simulink library "pv_sapm"  (R2018b)
settings: Solver=VariableStepAuto  StartTime=0.0  StopTime=10.0  RelTol=1e-3
undefined symbols (not defined in the file): Davies, Hay, path_carnot
libraries: carnot x4
settings Model: Creator=P41573  LastModifiedBy=P41573
settings SFSimCC: SimUseLocalCustomCode=off
settings RTWCC: RTWUseLocalCustomCode=off
settings CodeAppCC: StateflowObjectComments=on

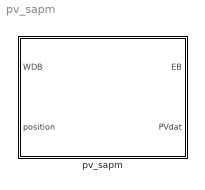
== system pv_sapm ==
  pv_sapm : Subsystem  mask(configurated PV Panel){PathName=fullfile(path_carnot('libsl'), 'Source', 'Electric_Generator', 'Pv_Sapm', 'parameter_set'), FileName='SandiaModuleDatabase.mat', Module=Yingli Solar YL230-29b Module - Sandia measured, userPath=on, userParam=off, Isco=8.222, Impo=7.727, Vmpo=29.886, Voco=37.28, T0=25, aIsc=0.000746, aImp=0.000176, BVoco=-0.1294, BVmpo=-0.137, n=1.263, SeriesCells=60, mBVoc=0, mBVmp=0, Ixo=8.1509, Ixxo=5.5099, C0=0.9993, C1=0.0007, C2=-0.058706, C3=-8.35334, C4=0.995, C5=0.005, C6=1.1325, C7=-0.1325, KbAngles=[0:5:90], Kb=[1 1 0.9999 0.9996 0.9991 0.9982 0.9965 0.9935 0.9886 0.9807 0.9678 0.9473 0.9148 0.8638 0.7846 0.6644 0.4907 0.2599 0], Kd=0.91, TypeMount=<propagated>, E0=1000, dTc=3, a=-3.348, b=-0.09143, TimeConstant=300, tini=20, ms=1, mp=1}
      mask prompts: PathName "Path"; FileName "DataBase"; Module "Parameter Set"; userPath "Edit path and name of parameter set"; userParam "User defined parameters"; Isco "reference short circuit current [A]"; Impo "reference maximum power point current [A]"; Vmpo "reference maximum power point voltage [V]"; Voco "reference open circuit voltage [V]"; T0 "reference cell temperature [°C]"; aIsc "temperature coef. for Isc [1/K]"; aImp "temperature coeff. for Imp [1/K]"; BVoco "temperature coef. for Voc [V/K]"; BVmpo "temperature coef. for Vmp [V/K]"; n "diode factor [n]"; SeriesCells "number of cells in series [-]"; mBVoc "irradiance dependant temperature coef. for Voc [V/K.wm2]"; mBVmp "irradiance dependant temperature coef. for Vmp [V/K.wm2]"; Ixo "Ix0 [A]"; Ixxo "Ixx0 [A]"; KbAngles "Kb: angles for longitudinal and transversal IAM [degree]"; Kb "Kb : incident angle modifier beam radiation"; Kd "Kd : Incidence angle modifier diffuse radiation"; TypeMount "Panel type / Mounting Option"; E0 "Reference Irradiation for deltaT (W/m2)"; dTc "SAPM parameter - deltaT [K]"; a "SAPM parameter - a [1]"; b "SAPM parameter - b [s/m]"; TimeConstant "time constant of sensor [s] - (not used)"; tini "initial cell temperature [°C] - (not used)"; ms "Number of modules in series"; mp "Number of modules in parallel"
      mask help:
      | PVPMC (PV-Lib) Single Diode equivalent Model with Sandia temperature model.
      | Parameter tables according to Sandia Module Database.
      mask init:
      | %%%%%%%%%%%%%%%%%[ok, param] = CarnotCallbacks_PvSapmConf('SetParameters',gcbh,PathName,FileName);
      mask Help: web(fullfile(path_carnot('help'),'pv_sapm.html'),'-helpbrowser')
      mask TypeOptions Module: <user defined> | 12-PW1000(95W)-Array - Sandia measured | 16-SanyoH552BA2-Array - Sandia measured | 32-BP380-Array - Sandia measured | 48-BP270 (70W)-Array - Sandia measured | 8 Sharp 167U1F Array - Sandia measured | 80-AstroPower AP75-Array - Sandia measured | 8-BP275-Array - Sandia measured | 8-KC80-Array - Sandia measured | 8-Shell Solar SM110-Array - Sandia measured | Advent Solar AS160 - Sandia measured | Advent Solar Ventura 210 - Sandia measured | Advent Solar Ventura 215 - Sandia measured | Aleo S03 160 | Aleo S03 165 | Aleo S16 165 | Aleo S16 170 | Aleo S16 175 | Aleo S16 180 | Aleo S16 185 | AstroPower AP-100 - Sandia measured | AstroPower AP-100 | AstroPower AP-110 - Sandia measured | AstroPower AP-110 | AstroPower AP-120 - Sandia measured | AstroPower AP-120 | AstroPower AP-1206 - Sandia measured | AstroPower AP-130 - Sandia measured | AstroPower AP-130 | AstroPower AP-50 - Sandia measured | AstroPower AP-50 | AstroPower AP-65 | AstroPower AP-75 - Sandia measured | AstroPower AP-75 - Sandia measured | AstroPower AP-75 | AstroPower AP-8225 - Sandia measured | AstroPower APX-110-SL - Sandia measured | AstroPower APX-110-SL | AstroPower APX-120 - Sandia measured | AstroPower APX-120 | AstroPower APX-130 - Sandia measured | AstroPower APX-130 | AstroPower APX-140 | AstroPower APX-40 | AstroPower APX-45 - Sandia measured | AstroPower APX-45 | AstroPower APX-45 | AstroPower APX-50 | AstroPower APX-65 - Sandia measured | AstroPower APX-65 | AstroPower APX-75 | AstroPower APX-75-SC | AstroPower APX-90 | BP Solar BP2140S | BP Solar BP2150S | BP Solar BP270 | BP Solar BP275 | BP Solar BP3110 | BP Solar BP3115 | BP Solar BP3120 | BP Solar BP3125 | BP Solar BP3125 | BP Solar BP3135 | BP Solar BP3150 | BP Solar BP3160 | BP Solar BP3180N - Sandia measured | BP Solar BP3220N Module - Sandia measured | BP Solar BP3232G - Sandia measured | BP Solar BP340 | BP Solar BP350 | BP Solar BP365 | BP Solar BP365TS | BP Solar BP380 - Sandia measured | BP Solar BP380 | BP Solar BP380 | BP Solar BP380J Module - Sandia measured | BP Solar BP380J Module | BP Solar BP4150 | BP Solar BP4160 | BP Solar BP4170 | BP Solar BP4175 | BP Solar BP485 | BP Solar BP5130 | BP Solar BP580 | BP Solar BP580 | BP Solar BP585 - Sandia measured | BP Solar BP585 | BP Solar BP585 | BP Solar BP980 | BP Solar BP990 | BP Solar MSX110 | BP Solar MSX120 | BP Solar MSX60 | BP Solar MSX64 | BP Solar SX110 | BP Solar SX110S | BP Solar SX120 | BP Solar SX120S | BP Solar SX140 | BP Solar SX150 | BP Solar SX160 | BP Solar SX160B | BP Solar SX170B | BP Solar SX305 | BP Solar SX310 | BP Solar SX3130 | BP Solar SX3140 | BP Solar SX3150 | BP Solar SX3160 | BP Solar SX3190 | BP Solar SX3195 | BP Solar SX320 | BP Solar SX3200 | BP Solar SX330 | BP Solar SX340 | BP Solar SX350 | BP Solar SX365 | BP Solar SX375 | BP Solar SX380 | BP Solar SX55 | BP Solar SX60 | BP Solar SX70 | BP Solar SX75 | Canadian Solar CS5P-220M - Sandia measured | Entech 22X Concentrator - Sandia measured | EPV-40 - Sandia measured | Evergreen ES-180 | Evergreen ES-180-RL-T Module - Sandia measured | Evergreen ES-180-RL-T Module | Evergreen ES-190 | Evergreen ES-195 | First Solar FS-265 | First Solar FS-267 | First Solar FS-270 | First Solar FS-272 - Sandia measured | First Solar FS-272 | First Solar FS-275 | First Solar FS-45 - Sandia measured | First Solar FS-45 | First Solar FS-50 - Sandia measured | First Solar FS-50 | First Solar FS-50 | First Solar FS-55 | First Solar FS-55 | Kyocera Solar KC120-1 - Sandia measured | Kyocera Solar KC120-1 | Kyocera Solar KC125G | Kyocera Solar KC130TM | Kyocera Solar KC150 - Sandia measured | Kyocera Solar KC150 | Kyocera Solar KC158G | Kyocera Solar KC167G | Kyocera Solar KC35 | Kyocera Solar KC40 | Kyocera Solar KC40T | Kyocera Solar KC45 | Kyocera Solar KC50 | Kyocera Solar KC50T | Kyocera Solar KC60 | Kyocera Solar KC60 | Kyocera Solar KC65T | Kyocera Solar KC70 | Kyocera Solar KC80 - Sandia measured | Kyocera Solar KC80 | Kyocera Solar KC80 | Kyocera Solar KC85T | Kyocera Solar KD135GX-LP | Kyocera Solar KD180GX-LP | Kyocera Solar KD205GX-LP | Kyocera Solar KS10 | Kyocera Solar KS10 | Kyocera Solar KS12 | Kyocera Solar KS16 | Kyocera Solar KS20 | Kyocera Solar KS20 | Kyocera Solar KS5 | Kyocera Solar KS5 | Kyocera Solar PV110 | Kyocera Solar PV120 | Kyocera Solar PV65 | Kyocera Solar PV75 | Ligitek LM220 BB00 - Sandia measured | Misubishi PV-MF115UE4N | Misubishi PV-MF120UE4N | Misubishi PV-MF125UE4N | Misubishi PV-MF130UE4N | Misubishi PV-UE115MF5N | Misubishi PV-UE120MF5N | Misubishi PV-UE125MF5N | Misubishi PV-UE130MF5N | Mitsubishi PV-MF165EB3 - Sandia measured | Mitsubishi PV-MF165EB3 | Mitsubishi PV-MF170EB4 | Mitsubishi PV-MF170UD4 | Mitsubishi PV-MF175UD4 | Mitsubishi PV-MF180UD4 | Mitsubishi PV-MF185UD4 | Mitsubishi PV-UD175MF5 | Mitsubishi PV-UD180MF5 | Mitsubishi PV-UD185MF5 | Mitsubishi PV-UD190MF5 | Moser Baer MBPV 220 Module - Sandia measured | Moser Baer MBPV 220 Module | Photowatt PW100 | Photowatt PW1000 (100W/12V) | Photowatt PW1000 (100W/24V) | Photowatt PW1000 (105W/12V) | Photowatt PW1000 (105W/24V) | Photowatt PW1000 (24V) - Sandia measured | Photowatt PW1000 (90W/12V) | Photowatt PW1000 (90W/24V) | Photowatt PW1000 (95W/12V) | Photowatt PW1000 (95W/24V) | Photowatt PW1000-12V | Photowatt PW1000-24V | Photowatt PW1250 | Photowatt PW1650-12 | Photowatt PW1650-24 | Photowatt PW200-12V | Photowatt PW500-12V | Photowatt PW6-110 | Photowatt PW6-123 | Photowatt PW6-230-12V | Photowatt PW6-230-24 | Photowatt PW750 | Photowatt PW850-12V | Photowatt PWX100 | Photowatt PWX200 | Photowatt PWX500 - Sandia measured | Photowatt PWX500 (42W) | Photowatt PWX500 (47W) | Photowatt PWX500 (52W) | Photowatt PWX750 (70W) | Photowatt PWX750 (75W) | Photowatt PWX750 (80W) | PowerLight PL-210-QM-I | PowerLight PL-225-QM-I | Sanyo H168 - Sandia measured | Sanyo HIP-180BA3 | Sanyo HIP-180DA3 Bifacial | Sanyo HIP-186BA3 | Sanyo HIP-186DA1 Bifacial | Sanyo HIP-186DA3 Bifacial | Sanyo HIP-190BA2 - Sandia measured | Sanyo HIP-190BA2 | Sanyo HIP-190BA3 | Sanyo HIP-190BE11 | Sanyo HIP-190DA1 Bifacial | Sanyo HIP-190DA3 Bifacial | Sanyo HIP-195BA3 | Sanyo HIP-195BE11 | Sanyo HIP-195DA3 Bifacial | Sanyo HIP-200BA19 - Sandia measured | Sanyo HIP-200BA3 | Sanyo HIP-200BE11 | Sanyo HIP-200DA3 Bifacial | Sanyo HIP-205BA3 | Sanyo HIP-205NKHE1 | Sanyo HIP-210NKHE1 | Sanyo HIP-215HDE1 | Sanyo HIP-215NKHE1 | Sanyo HIP-220HDE1 | Sanyo HIP-225HDE1 | Sanyo HIP-2717 | Sanyo HIP-55172 | Sanyo HIP-6219 | Sanyo HIP-63S1 | Sanyo HIP-6751B - Sandia measured | Sanyo HIP-6751B | Sanyo HIP-Bifacial Prototype - Sandia measured | Sanyo HIP-H552BA2 - Sandia measured | Sanyo HIP-HO97 - Sandia measured | Sanyo HIP-HO97 | Sanyo HIP-J54BA2 | Schott Solar ASE-100-ATF/17 (100) | Schott Solar ASE-100-ATF/17 (85) | Schott Solar ASE-100-ATF/17 (92) | Schott Solar ASE-100-ATF/34 (100) | Schott Solar ASE-100-ATF/34 (85) | Schott Solar ASE-100-ATF/34 (92) | Schott Solar ASE-250-DGF/50 (250) | Schott Solar ASE-270-DGF/50 (260) | Schott Solar ASE-270-DGF/50 (270) | Schott Solar ASE-300-DGF/17 (265) | Schott Solar ASE-300-DGF/17 (285) | Schott Solar ASE-300-DGF/17 (300) | Schott Solar ASE-300-DGF/50 - Sandia measured | Schott Solar ASE-300-DGF/50 (265) | Schott Solar ASE-300-DGF/50 (280) | Schott Solar ASE-300-DGF/50 (285) | Schott Solar ASE-300-DGF/50 (290) | Schott Solar ASE-300-DGF/50 (300) | Schott Solar ASE-300-DGF/50 (300) | Schott Solar ASE-300-DGF/50 (310) | Schott Solar ASE-300-DGF/50 (320) | Schott Solar ASE-50-ALF/17 - Sandia measured | Schott Solar ASE-50-ATF/17 (45) | Schott Solar ASE-50-ATF/17 (50) | Schott Solar SAPC 165 - Sandia measured | Schott Solar SAPC 165 | Schott Solar SAPC 170 | Schott Solar SAPC 175 | Sharp ND-070ERU/LU | Sharp ND-123U1 | Sharp ND-160E1 | Sharp ND-167U1 | Sharp ND-167U1F - Sandia measured | Sharp ND-167U1F | Sharp ND-187U1F | Sharp ND-208U1 | Sharp ND-208U1F | Sharp ND-216U1F | Sharp ND-216U2 | Sharp ND-L3E1U | Sharp ND-L3E6E | Sharp ND-NOECU | Sharp ND-Q0E2U | Sharp NE-165U1 | Sharp NE-170U1 | Sharp NE-80E1U | Sharp NE-H120E1 - Sandia measured | Sharp NE-H120E1 | Sharp NE-K125U2 | Sharp NE-Q5E2U | Sharp NT-175U1 | Sharp NT-185U1 | Sharp NT-5AE3D - Sandia measured | Sharp NT-R5E1U | Sharp NT-S5E1U | Shell Solar S10 | Shell Solar S105 | Shell Solar S115 | Shell Solar S165 - Sandia measured | Shell Solar S25 | Shell Solar S36 | Shell Solar S65 | Shell Solar S70-C | Shell Solar S75-C | Shell Solar S80 - Sandia measured | Shell Solar SM10 | Shell Solar SM100-12 | Shell Solar SM100-24 | Shell Solar SM110-12 | Shell Solar SM110-24 | Shell Solar SM20 | Shell Solar SM46 | Shell Solar SM50 | Shell Solar SM50-H | Shell Solar SM55 - Sandia measured | Shell Solar SM55 | Shell Solar SM6 - Sandia measured | Shell Solar SM6 | Shell Solar SP130 - Sandia measured | Shell Solar SP130 | Shell Solar SP140 | Shell Solar SP140 | Shell Solar SP150 | Shell Solar SP150 | Shell Solar SP18 (12V) | Shell Solar SP18 (6V) | Shell Solar SP36 (12V) | Shell Solar SP36 (6V) | Shell Solar SP65 (12V) | Shell Solar SP70 (12V) | Shell Solar SP70 (6V) | Shell Solar SP75 - Sandia measured | Shell Solar SP75 (12V) | Shell Solar SP75 (6V) | Shell Solar SQ140-PC | Shell Solar SQ150-PC | Shell Solar SQ160-PC | Shell Solar SQ70 <12V> | Shell Solar SQ70 <6V> | Shell Solar SQ75 <12V> | Shell Solar SQ75 <6V> | Shell Solar SQ80 <12V> | Shell Solar SQ80 <6V> | Shell Solar SR100 (12V) | Shell Solar SR100 (6V) | Shell Solar SR50 (12V) | Shell Solar SR50 (6V) | Shell Solar SR90 (12V) - Sandia measured | Shell Solar SR90 (12V) | Shell Solar SR90 (6V) | Shell Solar ST10 - Sandia measured | Shell Solar ST10 | Shell Solar ST20 | Shell Solar ST36 | Shell Solar ST40 | Shell Solar ST5 - Sandia measured | Shell Solar ST5 | Siemens Solar SM10 | Siemens Solar SM20 | Siemens Solar SM46 | Siemens Solar SM50 | Siemens Solar SM50-H | Siemens Solar SM55 - Sandia measured | Siemens Solar SM55 | Siemens Solar SM6 - Sandia measured | Siemens Solar SM6 | Siemens Solar SP130 - Sandia measured | Siemens Solar SP130 | Siemens Solar SP140 | Siemens Solar SP140 | Siemens Solar SP150 | Siemens Solar SP150 | Siemens Solar SP18 (12V) | Siemens Solar SP18 (6V) | Siemens Solar SP36 (12V) | Siemens Solar SP36 (6V) | Siemens Solar SP65 (12V) | Siemens Solar SP70 (12V) | Siemens Solar SP70 (6V) | Siemens Solar SP75 - Sandia measured | Siemens Solar SP75 (12V) | Siemens Solar SP75 (6V) | Siemens Solar SR100 (12V) | Siemens Solar SR100 (6V) | Siemens Solar SR50 (12V) | Siemens Solar SR50 (6V) | Siemens Solar SR90 (12V) - Sandia measured | Siemens Solar SR90 (12V) | Siemens Solar SR90 (6V) | Siemens Solar ST10 - Sandia measured | Siemens Solar ST10 | Siemens Solar ST20 | Siemens Solar ST40 | Siemens Solar ST5 - Sandia measured | Siemens Solar ST5 | Solar Fabrik SF-100 - Sandia measured | Solar Fabrik SF-115 - Sandia measured | Solar Semiconductor Inc. SSI-M6-220 Module - Sandia measured | Solar Semiconductor Inc. SSI-M6-220 Module | Solar World SW175 Mono Sun Module - Sandia measured | Solar World SW175 Mono Sun Module | Solarex MST-43LV - Sandia measured | Solarex MST-43LV | Solarex MST-43MV - Sandia measured | Solarex MST-43MV | Solarex MSX-110 | Solarex MSX-120 | Solarex MSX-120 | Solarex MSX-240 | Solarex MSX-60 | Solarex MSX-64 - Sandia measured | Solarex MSX-64 | Solarex MSX-64 (SiNx Proto) - Sandia measured | Solarex MSX-77 | Solarex MSX-83 | SolarFun SF220-30-P220 - Sandia measured | SolFocus SF-1100S-CPV-28 (315) | SolFocus SF-1100S-CPV-28 (330) | Suniva Titan 230 | Suniva Titan 240 | SunPower 128-Cell Module - Sandia measured | SunPower 128-Cell Module | SunPower 72 Cell prototype - Sandia measured | SunPower SP305 GEN C Module - Sandia measured | SunPower SP305 GEN C Module | SunPower SPR-200-BLK | SunPower SPR-200-BLK-U Module - Sandia measured | SunPower SPR-200-BLK-U Module | SunPower SPR-205-BLK | SunPower SPR-210-BLK | SunPower SPR-210-WHT - Sandia measured | SunPower SPR-210-WHT | SunPower SPR-210-WHT | SunPower SPR-210-WHT-U Module - Sandia measured | SunPower SPR-210-WHT-U Module | SunPower SPR-215-WHT | SunPower SPR-220 (CS) - Sandia measured | SunPower SPR-220 (PVL) - Sandia measured | SunPower SPR-220-BLK-U Module - Sandia measured | SunPower SPR-220-BLK-U Module | SunPower SPR-225-BLK | SunPower SPR-225-WHT | SunPower SPR-230-WHT | SunPower SPR-300-WHT | SunPower SPR-305-WHT - Sandia measured | SunPower SPR-305-WHT | SunPower SPR-315E-WHT | SunPower SPR-90 | SunPower SunTile | Suntech STP170S-24/Ac | Suntech STP175S-24/Ac | Suntech STP180S-24/Ac | Suntech STP200S-18/ub-1 Module - Sandia measured | Suntech STP200S-18/ub-1 Module | Suntech STP260S-24/Vb | Suntech STP270S-24/Vb | Suntech STP270S-24/Vb Module - Sandia measured | Suntech STP270S-24/Vb Module | Suntech STP280S-24/Vb | Uni-Solar PVL-116 | Uni-Solar PVL-124 | Uni-Solar PVL-128 | Uni-Solar PVL-136 | Uni-Solar PVL-29 | Uni-Solar PVL-58 | Uni-Solar PVL-64 | Uni-Solar PVL-68 | Uni-Solar PVL-87 | Uni-Solar SHR-17 | Uni-Solar US-11 | Uni-Solar US-116 | Uni-Solar US-21 | Uni-Solar US-3 | Uni-Solar US-32 - Sandia measured | Uni-Solar US-32 | Uni-Solar US-32 | Uni-Solar US-42 | Uni-Solar US-5 | Uni-Solar US-64 - Sandia measured | Uni-Solar US-64 | Uni-Solar US-64 | Uni-Solar USF-11 | Uni-Solar USF-32 | Uni-Solar USF-5 | Yingli Solar YL220 Module - Sandia measured | Yingli Solar YL220 Module | Yingli Solar YL230-29b Module - Sandia measured | Yingli Solar YL230-29b Module | Yingli YL210
      mask Callback Module: [ok, param] = CarnotCallbacks_PvSapm('SetParameters',gcbh);
      mask Callback userPath: [ok, param] = CarnotCallbacks_PvSapm('UserEdit',gcbh);
      mask Callback userParam: [ok, param] = CarnotCallbacks_PvSapm('UserEdit',gcbh);
      mask TypeOptions Isco: pvl_SAPM/Isc0
      mask TypeOptions Impo: pvl_SAPM/Imp0
      mask TypeOptions Vmpo: pvl_SAPM/Vmp0
      mask TypeOptions Voco: pvl_SAPM/Voc0
      mask TypeOptions T0: pvl_SAPM/T0
      mask TypeOptions aIsc: pvl_SAPM/AlphaIsc
      mask TypeOptions aImp: pvl_SAPM/AlphaImp
      mask TypeOptions BVoco: pvl_SAPM/BetaVoc
      mask TypeOptions BVmpo: pvl_SAPM/BetaVmp
      mask TypeOptions n: pvl_SAPM/n
      mask TypeOptions SeriesCells: pvl_SAPM/Ns
      mask TypeOptions mBVoc: pvl_SAPM/mBetaVoc
      mask TypeOptions mBVmp: pvl_SAPM/mBetaVmp
      mask TypeOptions Ixo: pvl_SAPM/Ix0
      mask TypeOptions Ixxo: pvl_SAPM/Ixx0
      mask TypeOptions C0: pvl_SAPM/c0
      mask TypeOptions C1: pvl_SAPM/c1
      mask TypeOptions C2: pvl_SAPM/c2
      mask TypeOptions C3: pvl_SAPM/c3
      mask TypeOptions C4: pvl_SAPM/c4
      mask TypeOptions C5: pvl_SAPM/c5
      mask TypeOptions C6: pvl_SAPM/c6
      mask TypeOptions C7: pvl_SAPM/c7
      mask TypeOptions KbAngles: IAM_Table/angle
      mask TypeOptions Kb: IAM_Table/Kb
      mask TypeOptions Kd: IAM_Table/Kd
      mask TypeOptions TypeMount: <propagated> | Glass/cell/glass - Open rack | Glass/cell/glass - Close roof mount | Glass/cell/polymer sheet - Open rack | Glass/cell/polymer sheet - Insulated back | Polymer/thin-film/steel - Open rack
      mask Callback TypeMount: [ok, param] = CarnotCallbacks_PvSapm('SetParameters',gcbh);
      mask DialogControl ParameterGroupVar Prompt: Picking a parameter set
      mask DialogControl Control2 Prompt: Carnot public data
      mask DialogControl Control2 Callback: [ok, file] = CarnotCallbacks_PvSapm('GetFilename',gcbh,'public');
      mask DialogControl Control3 Prompt: Carnot internal data
      mask DialogControl Control3 Callback: [ok, file] = CarnotCallbacks_PvSapm('GetFilename',gcbh,'internal');
      mask DialogControl Control4 Prompt: Selected path
      mask DialogControl Control4 Callback: [ok, file] = CarnotCallbacks_PvSapm('GetFilename',gcbh,'selected');
      mask DialogControl Container4 Prompt: Model Parameters
      mask DialogControl Container10 Prompt: Standard PV Parameters
      mask DialogControl Container12 Prompt: Detail Parameters
      mask DialogControl Container9 Prompt: Optics
      mask DialogControl Container14 Prompt: Temperature Model
      mask DialogControl Container15 Prompt: Array
      mask Display:
      | % user defined picture file
      | picfile = fullfile(path_carnot('intlibsl'), ...
      |         'Source','Electric_Generator','pv_sapm','parameter_set', ...
      |         'pv_sapm.jpg');
      | pic = false;
      | if ~BlockIsInCarnotLibrary    % if not located in library any more
      |     if exist(picfile,'file') % show internal picture if defined
      |         image(imread(picfile), [0.2, 0, 0.6, 1])
      |         set_param(gcb, 'BackgroundColor', 'White')
      |         pic = true;
      |     end
      | end
      | if ~pic    % show public picture
      |     disp('PV-Model\nSAPM')
      |     set_param(gcb, 'BackgroundColor', '[0.5,0.5,1]')%purple
      | end

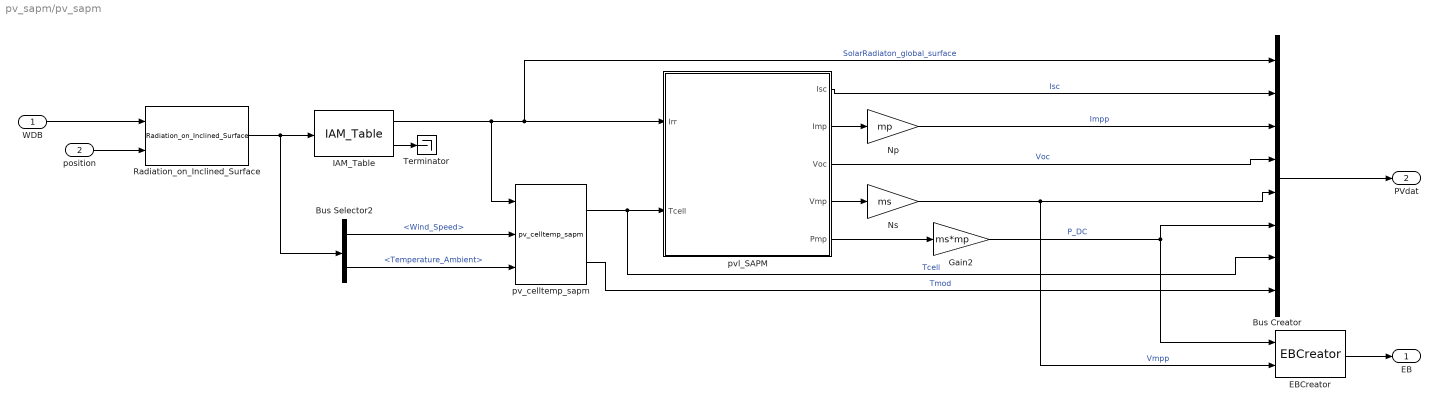
== system pv_sapm/pv_sapm ==
  WDB : Inport
  position : Inport  Port=2
  Bus Creator : BusCreator  Inputs=8
  Bus Selector2 : BusSelector  OutputSignals=Wind_Speed,Temperature_Ambient
  EBCreator : carnot/Basic/Electric/EBCreator  Inport_ID=off  Inport_f=off  Inport_v1=on  Inport_p1=on  Inport_pf1=off  Inport_v2=off  Inport_p2=off  Inport_pf2=off  Inport_v3=off  Inport_p3=off  Inport_pf3=off  ID=2  f=0  v1=0  p1=1e5  pf1=1  v2=0  p2=0  pf2=0  v3=0  p3=0  pf3=0  Annotation_ID=off  Annotation_f=off  Annotation_v1=off  Annotation_p1=off  Annotation_pf1=off  Annotation_v2=off  Annotation_p2=off  Annotation_pf2=off  Annotation_v3=off  Annotation_p3=off  Annotation_pf3=off
      settings: SourceProductName=Carnot
  Gain2 : Gain  Gain=ms*mp
  IAM_Table : carnot/Source/Solar_Thermal/IncidenceAngleModifier/IAM_Table  fta=1  angle=KbAngles  Kb=Kb  Kd=Kd
      settings: SourceProductName=Carnot
  Np : Gain  Gain=mp
  Ns : Gain  Gain=ms
  Radiation_on_Inclined_Surface : carnot/Weather/Radiation_on_Inclined_Surface  sky=Hay-Davies  reflect=0.2
      settings: SourceProductName=Carnot
  Terminator : Terminator
  pv_celltemp_sapm : carnot/Source/Electric_Generator/pv_celltemp_sapm  E0=1000  a=-3.47  b=-0.0594  dTc=2  TypeMount=Glass/cell/glass - Open rack  tini=25
      settings: SourceProductName=Carnot
  pvl_SAPM : MATLAB Function  TreatAsAtomicUnit=on  mask{Isc0=Isco, Imp0=Impo, Vmp0=Vmpo, Voc0=Voco, T0=T0, AlphaIsc=aIsc, AlphaImp=aImp, BetaVoc=BVoco, BetaVmp=BVmpo, mBetaVoc=mBVoc, mBetaVmp=mBVmp, Ix0=Ixo, Ixx0=Ixxo, n=n, Ns=SeriesCells, c0=C0, c1=C1, c2=C2, c3=C3, c4=C4, c5=C5, c6=C6, c7=C7}
      mask prompts: Isc0 "reference short circuit current [A]"; Imp0 "reference maximum power point current [A]"; Vmp0 "reference maximum power point voltage [V]"; Voc0 "reference open circuit voltage [V]"; T0 "reference cell temperature [°C]"; AlphaIsc "temperature coef. for Isc [1/K]"; AlphaImp "temperature coeff. for Imp [1/K]"; BetaVoc "temperature coef. for Voc [V/K]"; BetaVmp "temperature coef. for Vmp [V/K]"; mBetaVoc "irradiance dependant temperature coef. for Voc [V/K.wm2]"; mBetaVmp "irradiance dependant temperature coef. for Vmp [V/K.wm2]"; Ix0 "Ix0 [A]"; Ixx0 "Ixx0 [A]"; n "diode factor [n]"; Ns "number of cells in series [-]"
      mask init:
      | % alpha_isc = panel.alpha_sc;
      | % a_ref = panel.a_ref;
      | % IL_ref = panel.IL_ref;
      | % I0_ref = panel.I0_ref;
      | % Rsh_ref = panel.Rsh_ref;
      | % Rs_ref = panel.Rs_ref;
      | % Sref = panel.Sref;
      | % Tref = panel.Tref;
      | % EgRef = panel.EgRef;
      | % dEgdT = panel.dEgdT;
  EB : Outport
  PVdat : Outport  Port=2
  wires:
  IAM_Table/2 -> Terminator/1
  pv_celltemp_sapm/1 -> Bus Creator/7, pvl_SAPM/2(Tcell)  "Tcell"
  Bus Selector2/1 -> pv_celltemp_sapm/2  "<Wind_Speed>"
  pvl_SAPM/1(Isc) -> Bus Creator/2  "Isc"
  pvl_SAPM/2(Imp) -> Np/1
  pvl_SAPM/5(Pmp) -> Gain2/1
  pv_celltemp_sapm/2 -> Bus Creator/8  "Tmod"
  Bus Selector2/2 -> pv_celltemp_sapm/3  "<Temperature_Ambient>"
  WDB/1 -> Radiation_on_Inclined_Surface/1
  position/1 -> Radiation_on_Inclined_Surface/2
  Ns/1 -> Bus Creator/5, EBCreator/2  "Vmpp"
  Np/1 -> Bus Creator/3  "Impp"
  pvl_SAPM/4(Vmp) -> Ns/1
  pvl_SAPM/3(Voc) -> Bus Creator/4  "Voc"
  Radiation_on_Inclined_Surface/1 -> Bus Selector2/1, IAM_Table/1
  EBCreator/1 -> EB/1
  Bus Creator/1 -> PVdat/1
  IAM_Table/1 -> pv_celltemp_sapm/1, Bus Creator/1, pvl_SAPM/1(Irr)  "SolarRadiaton_global_surface"
  Gain2/1 -> EBCreator/1, Bus Creator/6  "P_DC"

== matlab function pv_sapm/pvl_SAPM ==
  data: Isc output; Imp output; Voc output; Vmp output; Irr input size=1; Tcell input size=1; Ix0 parameter; Pmp output; AlphaIsc parameter; AlphaImp parameter; Voc0 parameter; BetaVoc parameter; mBetaVoc parameter; BetaVmp parameter size=1; mBetaVmp parameter size=1; n parameter size=1; Ns parameter size=1; Isc0 parameter size=1; C0 parameter; Ixx0 parameter; Vmp0 parameter; Imp0 parameter; C1 parameter; C2 parameter; C3 parameter; C4 parameter; C5 parameter; C6 parameter; C7 parameter
function [Isc, Imp, Voc, Vmp, Pmp] = pvl_sapm(Irr, Tcell, Ix0, AlphaIsc, AlphaImp,...
                                                        Voc0, BetaVoc, mBetaVoc, BetaVmp, mBetaVmp, n, Ns, Isc0,...
                                                        C0, Ixx0, Vmp0, Imp0, C1, C2, C3, C4, C5, C6, C7)

%% PVL_SAPM Performs Sandia PV Array Performance Model to get 5 points on IV curve given SAPM module parameters, Ee, and cell temperature
%
% Syntax
%   Result = pvl_sapm(Module, Ee, celltemp)
%
% Description
%   The Sandia PV Array Performance Model (SAPM) generates 5 points on a PV
%   module's I-V curve (Voc, Isc, Ix, Ixx, Vmp/Imp) according to
%   SAND2004-3535. Assumes a reference cell temperature of 25 C.
% Inputs
%   Module - a structure defining the SAPM performance parameters (see
%   below)
%   Ee - The effective irradiance incident upon the module (suns). Any Ee<0
%   are set to 0.
%   celltemp - The cell temperature (degrees C)
% Outputs
%   Result - A structure with Result.Isc, Result.Imp, Result.Ix,
%   Result.Ixx, Result.Voc, Result.Vmp, and Result.Pmp. Structure
%   components are vectors of the same size as Ee.
%
% Note - The particular coefficients from SAPM which are required in Module
% are:
%   Module.c - 1x8 vector with the C coefficients Module.c(1) = C0
%   Module.Isc0 - Short circuit current at reference condition (amps)
%   Module.Imp0 - Maximum power current at reference condition (amps)
%   Module.AlphaIsc - Short circuit current temperature coefficient at
%     reference condition (1/C)
%   Module.AlphaImp - Maximum power current temperature coefficient at
%     reference condition (1/C)
%   Module.BetaVoc - Open circuit voltage temperature coefficient at
%     reference condition (V/C)
%   Module.mBetaVoc - Coefficient providing the irradiance dependence for
%     the BetaVoc temperature coefficient at reference irradiance (V/C)
%   Module.BetaVmp - Maximum power voltage temperature coefficient at
%     reference condition
%   Module.mBetaVmp - Coefficient providing the irradiance dependence for
%     the BetaVmp temperature coefficient at reference irradiance (V/C)
%   Module.n - Empirically determined "diode factor" (dimensionless)
%   Module.Ns - Number of cells in series in a module's cell string(s)
%
% References
%   [1] King, D. et al, 2004, "Sandia Photovoltaic Array Performance Model", SAND Report
%   3535, Sandia National Laboratories, Albuquerque, NM
%
% See also PVL_SAPMMODULEDB PVL_SAPMCELLTEMP 



%% normalize Irradiation
Irr = Irr/1000;
% Make sure inputs are of the same size
if size(Irr) ~= size(Tcell)
    error('Error in pvl_sapm. celltemp and Ee must be vectors of the same size')
end

%   Define Constants
Const.T0 = 25;          %Reference temperature (25 deg C)
Const.q = 1.60218E-19;  %Elementary charge (1.60218E-19 coulombs
Const.k = 1.38066E-23;  %Boltzmann's constant (1.38066E-23 J/K)

% Create output variables, set them to 0
Isc = 0*Irr;
Imp = 0*Irr;
Voc = 0*Irr;
Vmp = 0*Irr;
Ix = 0*Irr;
Ixx = 0*Irr;
Pmp = 0*Irr;

% Create other variables, set them to 0
delta = 0*Irr;
BetaVocRes = 0*Irr;
BetaVmpRes = 0*Irr;
Irr(Irr<0) = 0;
filter = (Irr >= 1e-3); % Don't perform SAPM on Ee values < 1E-3

Isc(filter) = Isc0 .* Irr(filter) .* (1+AlphaIsc .*(Tcell(filter) - Const.T0));
Imp(filter) = Imp0.*(C0.* Irr(filter) + C1*(Irr(filter).^2)).*(1 + AlphaImp .* (Tcell(filter) - Const.T0));
BetaVocRes(filter) = BetaVoc + mBetaVoc .* (1-Irr(filter));
delta(filter) = n .* Const.k .* (Tcell(filter) + 273.15) ./ Const.q;
Voc(filter) = (Voc0 + Ns .* delta(filter) .* log(Irr(filter)) + BetaVocRes(filter) .* (Tcell(filter) - Const.T0));
BetaVmpRes(filter) = BetaVmp + mBetaVmp .* (1-Irr(filter));
Vmp(filter) = (Vmp0 + C2 .* Ns .* delta(filter) .* log(Irr(filter))+ C3 .* Ns .* (delta(filter) .* log(Irr(filter))).^2 + BetaVmpRes(filter) .* (Tcell(filter) - Const.T0));
Pmp = Imp .* Vmp;
Ix(filter) = Ix0*(C4 .* Irr(filter) + C5 .* (Irr(filter)).^2) .*...
    (1 + AlphaIsc.*(Tcell(filter)-Const.T0));
Ixx(filter) = Ixx0*(C6 .* Irr(filter) + C7 .* (Irr(filter)).^2) .*...
    (1 + AlphaIsc.*(Tcell(filter)-Const.T0));
